simulink model "DSimulator_robot3GDL"  (Simulink 10.1)
settings: Solver=ode1  StartTime=0  StopTime=200  FixedStep=0.004  RelTol=1e-3  EnableMultiTasking=on
undefined symbols (not defined in the file or in its folder): Dinamic_ur10_3DOF, SimpleRobotPlotROS, Tau, TrajGen
libraries: simulink x6
settings Model: Creator=E. Dean  LastModifiedBy=tard
settings DataIOCC: LimitDataPoints=on  SignalLoggingSaveFormat=ModelDataLogs
settings OptimizationCC: ExpressionDepthLimit=2147483647
settings DebuggingCC: SolverPrmCheckMsg=warning  FcnCallInpInsideContextMsg=warning  AllowSymbolicDim=off  StateNameClashWarn=warning
settings ConfigComp: CovSFcnEnable=off

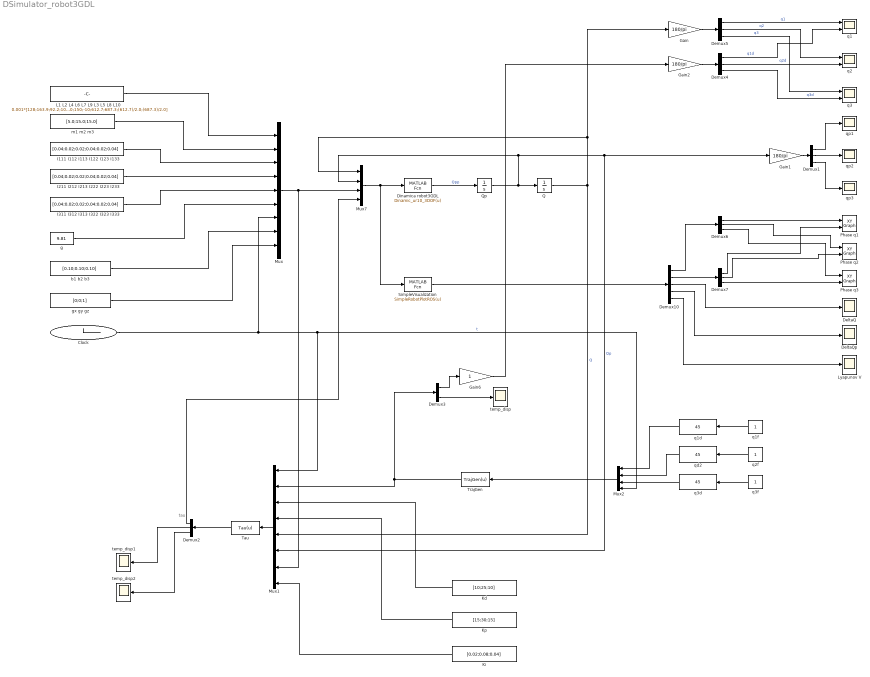
== system DSimulator_robot3GDL ==
  note: tau
  Clock : Clock
  DeltaQ : Scope
  DeltaQp : Scope
  Demux{1..2,4..7} (6 alike) : Demux  Outputs=3
  Demux10 : Demux  Outputs=5
  Demux3 : Demux  Outputs=2
  Dinamica robot3GDL : MATLABFcn  MATLABFcn=Dinamic_ur10_3DOF(u)  OutputDimensions=3
  Gain : Gain  Gain=180/pi
  Gain1 : Gain  Gain=180/pi
  Gain2 : Gain  Gain=180/pi
  Gain6 : Gain
  I111 I112 I113 I122 I123 I133 : Constant  Value=[0.04;0.02;0.02;0.04;0.02;0.04]
  I211 I212 I213 I222 I223 I233 : Constant  Value=[0.04;0.02;0.02;0.04;0.02;0.04]
  I311 I312 I313 I322 I323 I333 : Constant  Value=[0.04;0.02;0.02;0.04;0.02;0.04]
  "Kd " : Constant  Value=[10;25;10]
  Ki : Constant  Value=[0.02;0.08;0.04]
  Kp : Constant  Value=[15;30;15]
  "L1 L2 L4 L6 L7 L9 L3 L5 L8 L10 " : Constant  Value=0.001*[128;163.9;92.2;100;150;-10;612.7;687.3;(612.7)/2.0;(687.3)/2.0]  VectorParams1D=off
  Lyapunov V : Scope
  Mux : Mux  Inputs=9
  Mux1 : Mux  Inputs=8
  Mux2 : Mux
  Mux7 : Mux
  Phase q1 : simulink/Sinks/XY Graph  xmin=-pi  xmax=pi  ymin=-1  ymax=1  st=-1
  Phase q2 : simulink/Sinks/XY Graph  xmin=-pi  xmax=pi  ymin=-1  ymax=1  st=-1
  Phase q3 : simulink/Sinks/XY Graph  xmin=-pi  xmax=pi  ymin=-1  ymax=1  st=-1
  Q : Integrator  InitialCondition=[0;0;0]
  Qp : Integrator  InitialCondition=[0;0;0]
  SimpleVisualization : MATLABFcn  MATLABFcn=SimpleRobotPlotROS(u)  OutputDimensions=13
  "Tau " : MATLABFcn  MATLABFcn=Tau(u)  OutputDimensions=9
  TrajGen : MATLABFcn  MATLABFcn=TrajGen(u)  OutputDimensions=6
  "b1 b2 b3 " : Constant  Value=[0.10;0.10;0.10]
  g : Constant  Value=9.81
  gx gy gz : Constant  Value=[0;0;1]
  "m1 m2 m3 " : Constant  Value=[5.0;15.0;15.0]
  q1 : Scope  NumInputPorts=2
  q1d : simulink/Math Operations/Slider Gain  gain=45  low=-180  high=180
  q1f : Constant
  q2 : Scope  NumInputPorts=2
  q2f : Constant
  q3 : Scope  NumInputPorts=2
  q3d : simulink/Math Operations/Slider Gain  gain=45  low=-180  high=180
  q3f : Constant
  qd2 : simulink/Math Operations/Slider Gain  gain=45  low=-180  high=180
  qp1 : Scope
  qp2 : Scope
  qp3 : Scope
  temp_disp : Scope
  temp_disp1 : Scope
  temp_disp2 : Scope
  wires:
  Dinamica robot3GDL/1 -> Qp/1  "Qpp"
  Gain1/1 -> Demux1/1
  Demux1/1 -> qp1/1
  Demux1/2 -> qp2/1
  Demux1/3 -> qp3/1
  I111 I112 I113 I122 I123 I133/1 -> Mux/3
  I211 I212 I213 I222 I223 I233/1 -> Mux/4
  I311 I312 I313 I322 I323 I333/1 -> Mux/5
  "b1 b2 b3 "/1 -> Mux/8
  Mux1/1 -> "Tau "/1
  TrajGen/1 -> Demux3/1, Mux1/2
  q1f/1 -> q1d/1
  q2f/1 -> qd2/1
  q3f/1 -> q3d/1
  Mux2/1 -> TrajGen/1
  q1d/1 -> Mux2/1
  qd2/1 -> Mux2/2
  q3d/1 -> Mux2/3
  "Kd "/1 -> Mux1/3
  Kp/1 -> Mux1/4
  Q/1 -> Gain/1, Mux7/1, Mux1/5  "Q"
  Qp/1 -> Mux1/6, Gain1/1, Mux7/2, Q/1  "Qp"
  "Tau "/1 -> Demux2/1
  "m1 m2 m3 "/1 -> Mux/2
  g/1 -> Mux/6
  "L1 L2 L4 L6 L7 L9 L3 L5 L8 L10 "/1 -> Mux/1
  Clock/1 -> Mux/7, Mux2/4, Mux1/1  "t"
  Ki/1 -> Mux1/8
  Demux3/1 -> Gain6/1
  Demux4/1 -> q1/2  "q1d"
  Demux5/1 -> q1/1  "q1"
  Demux5/2 -> q2/1  "q2"
  Gain6/1 -> Gain2/1
  gx gy gz/1 -> Mux/9
  Demux5/3 -> q3/1  "q3"
  Demux4/2 -> q2/2  "q2d"
  Demux4/3 -> q3/2  "q3d"
  Demux2/2 -> temp_disp1/1
  Demux2/3 -> temp_disp2/1
  Demux3/2 -> temp_disp/1
  SimpleVisualization/1 -> Demux10/1
  Demux10/1 -> Demux6/1
  Demux10/2 -> Demux7/1
  Demux10/3 -> DeltaQ/1
  Demux10/4 -> DeltaQp/1
  Demux10/5 -> Lyapunov V/1
  Demux6/1 -> Phase q1/1
  Demux6/2 -> Phase q2/1
  Demux6/3 -> Phase q3/1
  Demux7/1 -> Phase q1/2
  Demux7/2 -> Phase q2/2
  Demux7/3 -> Phase q3/2
  Mux7/1 -> SimpleVisualization/1, Dinamica robot3GDL/1
  Mux/1 -> Mux7/3, Mux1/7
  Gain/1 -> Demux5/1
  Gain2/1 -> Demux4/1
  Demux2/1 -> Mux7/4
